simulink library "ZeroProtectionLibrary"  (R2015a)
settings: Solver=ode45  StartTime=0.0  StopTime=10.0  RelTol=1e-3
undefined symbols (not defined in the file or in its folder): Threshold
libraries: simulink x1
settings Model: Creator=Cam  LastModifiedBy=Cam

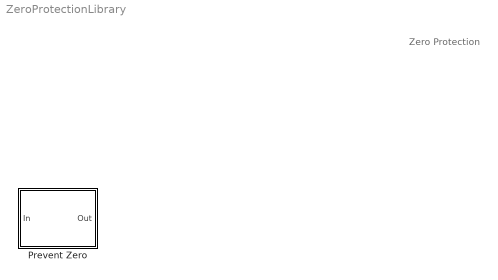
== system ZeroProtectionLibrary ==
  note: Zero Protection
  Prevent Zero : Subsystem  mask(Prevent Zero){thresh=0.1}
      mask prompts: thresh "Threshold:"
      mask help: Prevents the output from going to zero. When the absolute value of the input is less than the Threshold, replace the value with the signed version of the Threshold.
      mask Display: disp('Prevent\nZero')

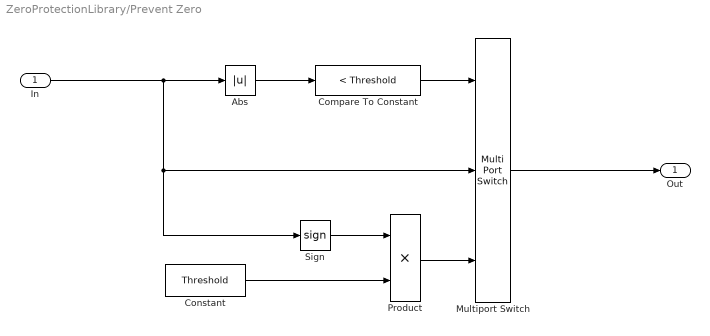
== system ZeroProtectionLibrary/Prevent Zero ==
  In : Inport
  Abs : Abs
  Compare To Constant : simulink/Logic and Bit Operations/Compare To Constant  relop=<  const=Threshold  OutDataTypeStr=boolean
  Constant : Constant  Value=Threshold
  Multiport Switch : MultiPortSwitch  DataPortOrder=Zero-based contiguous  Inputs=2
  Product : Product
  Sign : Signum
  Out : Outport
  wires:
  In/1 -> Sign/1, Multiport Switch/2, Abs/1
  Compare To Constant/1 -> Multiport Switch/1
  Multiport Switch/1 -> Out/1
  Product/1 -> Multiport Switch/3
  Constant/1 -> Product/2
  Sign/1 -> Product/1
  Abs/1 -> Compare To Constant/1
